simulink model "Ctrl_WT_openPI_IMC"  (R2019b)
settings: Solver=ode23tb  StartTime=0.0  StopTime=20  MaxStep=1/60  RelTol=1e-4  AbsTol=1e-3  EnableMultiTasking=on
InitFcn:
  | xInitial = init_power_wind_ig;
values from neighbouring files (symbols this model uses):
  GDes = tf(1,[0.2/n 1])^n    [lin_WT.m]
  GProc = zpk_min(1,1)    [lin_WT.m]
undefined symbols (not defined in the file or in its folder): D1, Delta, F, find_system, Fnom, gcbh, H, Llr, Lls, p, Pnom, Rr, Rs, sps_rtmsupport, Vnom
libraries: powerlib x14, cstblocks x13, powerlib_meascontrol x4, re_lib x1
settings Model: PauseTimes=15  ExtModeAutoUpdateStatusClock=off  Creator=MathWorks  LastModifiedBy=estuser04
settings SolverCC: AutoScaleAbsTol=off  SolverResetMethod=Robust
settings DataIOCC: LimitDataPoints=on  SaveFormat=Array  SignalLoggingSaveFormat=ModelDataLogs  SaveOutput=off  SaveTime=off  ReturnWorkspaceOutputs=off  SignalLoggingName=logsOut
settings OptimizationCC: BlockReduction=off  DefaultParameterBehavior=Inlined  BufferReuse=off  ExpressionDepthLimit=2147483647  InitFltsAndDblsToZero=on  LifeSpan=inf
settings DebuggingCC: UnderspecifiedInitializationDetection=Classic  MergeDetectMultiDrivingBlocksExec=none  CheckExecutionContextPreStartOutputMsg=on  CheckExecutionContextRuntimeOutputMsg=on  SignalResolutionControl=TryResolveAllWithWarning  SolverPrmCheckMsg=warning  MultiTaskDSMMsg=warning  MultiTaskCondExecSysMsg=none  FcnCallInpInsideContextMsg=warning  StateNameClashWarn=warning  InitInArrayFormatMsg=none  SFUnexpectedBacktrackingDiag=warning  SFNoUnconditionalDefaultTransitionDiag=warning  SFExecutionAtInitializationDiag=none  ArithmeticOperatorsInVariantConditions=warning
settings HardwareCC: ProdBitPerPointer=32  ProdBitPerSizeT=32  ProdBitPerPtrDiffT=32  ProdLargestAtomicFloat=None  ProdIntDivRoundTo=Undefined  ProdEndianess=Unspecified  ProdWordSize=32  ProdHWDeviceType=32-bit Generic
settings ModelReferenceCC: PropagateSignalLabelsOutOfModel=off
settings SFSimCC: SimUseLocalCustomCode=off  CustomCodeUndefinedFunction=UseInterfaceOnly
settings RTWCC: RTWUseLocalCustomCode=off
settings CodeAppCC: StateflowObjectComments=on
settings GRTTargetCC: TargetLangStandard=C89/C90 (ANSI)  GeneratePreprocessorConditionals=Disable all  CombineOutputUpdateFcns=off  GRTInterface=on
settings ConfigComp: CovMetricSettings=dw  CovHtmlReporting=on  CovSaveCumulativeToWorkspaceVar=on  CovSaveSingleToWorkspaceVar=on  CovExternalEMLEnable=off  CovSFcnEnable=off
settings SimscapeCC: SimscapeNormalizeSystem=off

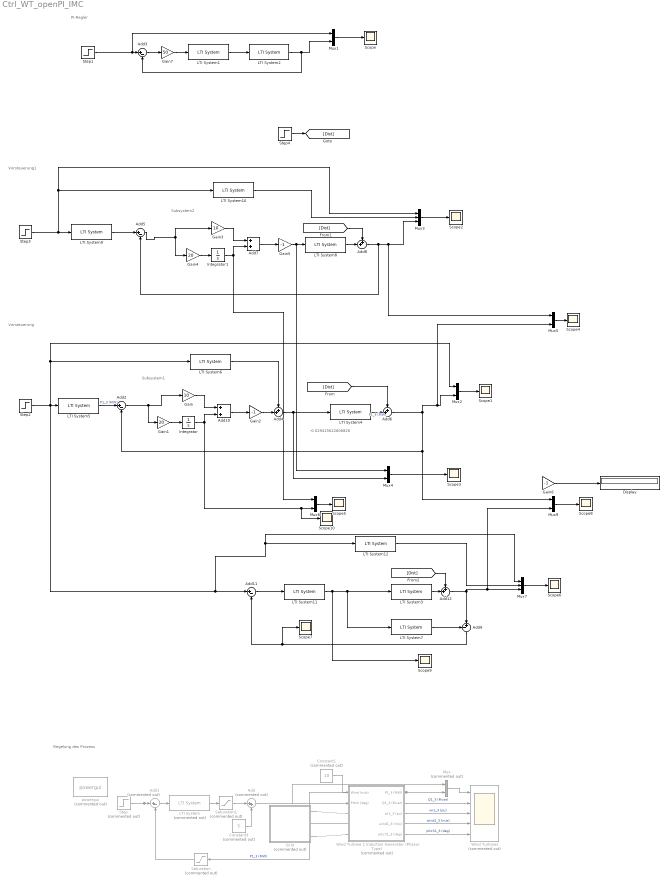
== system Ctrl_WT_openPI_IMC ==
  note: -0.029415622606826
  note: Subsystem2
  note: Subsystem1
  note: Regelung des Prozess
  note: PI-Regler
  note: Vorsteuerung
  note: Vorsteuerung1
  " Wind Turbines" : Scope  Commented=on  NumInputPorts=5
  Add : Sum  Commented=on  Inputs=|++
  Add1 : Sum  Commented=on  Inputs=|+-
  Add10 : Sum
  Add{2..3,5,11} (4 alike) : Sum  Inputs=|+-
  Add{4,6,8,12} (4 alike) : Sum  Inputs=++|
  Add7 : Sum
  Add9 : Sum  Inputs=-+|
  Constant1 : Constant  Commented=on  Value=10
  Constant3 : Constant  Commented=on  Value=5
  Display : Display
  Gain : Gain  Gain=10
  Gain1 : Gain  Gain=20
  Gain2 : Gain  Gain=-1
  Gain3 : Gain  Gain=10
  Gain4 : Gain  Gain=20
  Gain5 : Gain  Gain=-1
  Gain6 : Gain  Gain=-1
  Gain7 : Gain  Gain=50
  Grid : Subsystem  Commented=on
  Integrator : Integrator
  Integrator1 : Integrator
  LTI System : cstblocks/LTI System  Commented=on  sys=Creg  IC=[]
  LTI System1 : cstblocks/LTI System  sys=GRegPI  IC=[]
  LTI System10 : cstblocks/LTI System  sys=GDes  IC=[]
  LTI System11 : cstblocks/LTI System  sys=GDes/GProc  IC=[]
  LTI System12 : cstblocks/LTI System  sys=GDes  IC=[]
  LTI System2 : cstblocks/LTI System  sys=GProc  IC=[]
  LTI System{3..4,7..8} (4 alike) : cstblocks/LTI System  sys=GProcReal  IC=[]
  LTI System5 : cstblocks/LTI System  sys=GDes  IC=[]
  LTI System6 : cstblocks/LTI System  sys=GFF2  IC=[]
  LTI System9 : cstblocks/LTI System  sys=GFF  IC=[]
  Mux : Mux  Commented=on  Inputs=2
  Mux{1..2,4..6,9} (6 alike) : Mux  Inputs=2
  Mux3 : Mux  Inputs=3
  Mux7 : Mux  Inputs=3
  Saturation : Saturate  Commented=on  UpperLimit=1.5  LowerLimit=0.5
  Saturation1 : Saturate  Commented=on  UpperLimit=20  LowerLimit=-5
  Scope{,1..10} (11 alike) : Scope
  Step : Step  Commented=on  Time=5  Before=0.85  After=0.7  SampleTime=0
  Step1 : Step  Time=5  SampleTime=0
  Step2 : Step  Time=5  SampleTime=0
  Step3 : Step  Time=5  SampleTime=0
  Step4 : Step  Time=8  After=0  SampleTime=0
  Wind Turbine 1 Induction Generator (Phasor Type) : Subsystem  Commented=on  DialogController=POWERSYS.PowerSysDialog  LoadFcn=sps_rtmsupport('LoadFcn',gcbh); %find_system(gcs,'FollowLinks', 'on', 'LookUnderMasks', 'all');  StartFcn=sps_rtmsupport('StartFcn',gcbh);  StopFcn=sps_rtmsupport('StopFcn',gcbh);  mask(Wind Turbine Induction Generator (Phasor Type)){ExternalTm=off, nom=[2*1.5e6/0.9 575 60], sta=[ 0.004843 0.1248], rot=[ 0.004377 0.1791], Lm=6.77, mec=[5.04 0.01 3], init=[ -0.01,0   0,0,0   0,0,0 ], pitch_angle=0, Pmec=2*1.5e6, wind_base=9, speed_nom=1, P_wind_base=1, K_pitch_gain=[5 25], pitch_max=45, pitch_rate=2}
      mask prompts: ExternalTm "External turbine (Tm mechanical torque input)"; nom "Nominal power, line-to-line voltage, frequency [Pn(VA), Vn(Vrms), fn(Hz)]:"; sta "Stator [Rs, Lls] (pu):"; rot "Rotor [Rr', Llr'] (pu):"; Lm "Magnetizing inductance Lm (pu):"; mec "Inertia constant, friction factor, and pairs of poles: [H(s), F(pu), p]"; init "Initial conditions [s, th(deg), ias, ibs, ics (pu), ph_as, ph_bs, ph_cs (pu)]:"; pitch_angle "Pitch angle beta used to display characteristics (beta >=0)  (deg):"; Pmec "Nominal wind turbine mechanical output power (W):"; wind_base "Base wind speed (m/s):"; speed_nom "Base rotational speed (pu of base generator speed):"; P_wind_base "Maximum power at base wind speed (pu of nominal mechanical power):"; K_pitch_gain "Pitch angle controller gain: [Kp Ki]"; pitch_max "Maximum pitch angle (deg):"; pitch_rate "Maximum rate of change of pitch angle (deg/s):"
      mask help: Implements a phasor model of a squirrel-cage induction generator driven by a wind turbine.
      mask init:
      | [Pnom,Vnom,Fnom,Rs,Lls,Rr,Llr,H,p,F,Wind_On,FACTSroot] = WindTurbineIndGenInit (nom,sta,rot,mec,ExternalTm,wind_base,gcbh);
      settings: CopyFcn=sps_rtmsupport('CopyFcn',gcbh);  DeleteFcn=sps_rtmsupport('DeleteFcn',gcbh);  UndoDeleteFcn=sps_rtmsupport('UndoDeleteFcn',gcbh);  ModelCloseFcn=sps_rtmsupport('ModelCloseFcn',gcbh);  PreSaveFcn=sps_rtmsupport('PreSaveFcn',gcbh);  PostSaveFcn=sps_rtmsupport('PostSaveFcn',gcbh);  NameChangeFcn=sps_rtmsupport('NameChangeFcn',gcbh);  PreCopyFcn=sps_rtmsupport('PreCopyFcn',gcbh);  OpenFcn=sps_rtmsupport('OpenFcn',gcbh, [1]);  CloseFcn=sps_rtmsupport('CloseFcn',gcbh);  PreDeleteFcn=sps_rtmsupport('PreDeleteFcn',gcbh);
      mask Help: helpview(psbhelp);
      mask Callback ExternalTm: WindTurbineIndGenCback(gcbh);
      mask DialogControl generatordata Prompt: Generator
      mask DialogControl Turbine Prompt: Turbine
      mask DialogControl display Prompt: Display wind turbine power characteristics
      mask DialogControl display Callback: WindTurbineIndGenDisplay(gcbh);
  powergui : powerlib/powergui  Priority=2  Commented=on  SimulationMode=Phasor  SampleTime=0  frequency=60  Iterations=50  frequencyindice=60  Pbase=100e6  ErrMax=1e-4  UnitsV=kV  UnitsW=MW  buscounter=0  FunctionMessages=off  echomessages=off  EnableUseOfTLC=off  CurrentSourceSwitches=off  DisableSnubberDevices=off  DisableRonSwitches=off  DisableVfSwitches=off  DisplayEquations=off  AutomaticDiscreteSolvers=off  SolverType=Tustin  Interpol=off  ExternalGateDelay=off  methode=off  Ts=0  x0status=blocks  SPID=off  SwTol=0  HookPort=off  NonlinearTolerance=1e-4  nMaxIteration=100  ContinueOnMaxIteration=off  RestoreLinks=no  ResistiveCurrentMeasurement=off  Frange=[0:2:500]  Ylog=off  Xlog=off  ShowGrid=off  save=off  variable=ZData  structure=0  ZoomFFT=on  StartTime=0.0  cycles=1  DisplayStyle=1  fundamental=60  FreqAxis=off  MaxFrequency=1000  frequencyindicesteady=1  RmsSteady=1  display=off
      settings: SourceProductName=Simscape Electrical
  wires:
  Add/1 -> Wind Turbine 1 Induction Generator (Phasor Type)/2(Pitch (deg))
  Wind Turbine 1 Induction Generator (Phasor Type)/1(P1_3 (MW)) -> Mux/2, Saturation/1  "P1_3 (MW)"
  Wind Turbine 1 Induction Generator (Phasor Type)/4(wind1_3 (m/s)) -> " Wind Turbines"/4  "wind1_3 (m/s)"
  Wind Turbine 1 Induction Generator (Phasor Type)/3(wr1_3 (pu)) -> " Wind Turbines"/3  "wr1_3 (pu)"
  Constant1/1 -> Wind Turbine 1 Induction Generator (Phasor Type)/1("Wind (m/s) ")
  Wind Turbine 1 Induction Generator (Phasor Type)/2(Q1_3 (Mvar)) -> " Wind Turbines"/2  "Q1_3 (Mvar)"
  Wind Turbine 1 Induction Generator (Phasor Type)/5(pitch1_3 (deg)) -> " Wind Turbines"/5  "pitch1_3 (deg)"
  LTI System/1 -> Saturation1/1
  Add1/1 -> LTI System/1
  Saturation/1 -> Add1/2
  Step/1 -> Mux/1, Add1/1
  Saturation1/1 -> Add/1
  Constant3/1 -> Add/2
  Mux/1 -> " Wind Turbines"/1
  Mux1/1 -> Scope/1
  Step1/1 -> Add3/1, Mux1/1
  Add3/1 -> Gain7/1
  LTI System2/1 -> Mux1/2, Add3/2
  LTI System1/1 -> LTI System2/1
  LTI System4/1 -> Add6/2  "P1_3 (MW)"
  Mux2/1 -> Scope1/1
  LTI System5/1 -> Add2/1  "P1_3 (MW)"
  Gain2/1 -> Add4/2
  LTI System6/1 -> Add4/1
  Gain5/1 -> Mux4/1, LTI System8/1
  LTI System8/1 -> Add8/2
  Step3/1 -> LTI System9/1, LTI System10/1, Mux3/1
  Mux3/1 -> Scope2/1
  LTI System9/1 -> Add5/1
  LTI System10/1 -> Mux3/2
  Mux4/1 -> Scope3/1
  Add6/1 -> Mux9/1, Add2/2, Mux5/2, Mux2/2
  Add2/1 -> Gain1/1, Gain/1
  Integrator/1 -> Scope10/1, Mux6/2, Add10/2
  Add10/1 -> Gain2/1
  Gain/1 -> Add10/1
  Gain1/1 -> Integrator/1
  Gain4/1 -> Integrator1/1
  Gain3/1 -> Add7/1
  Add7/1 -> Gain5/1
  Integrator1/1 -> Mux6/1, Add7/2
  Add5/1 -> Gain4/1, Gain3/1
  Add8/1 -> Mux5/1, Mux3/3, Add5/2
  Step4/1 -> [Dist]
  [Dist] -> Add6/1
  [Dist] -> Add8/1
  Mux5/1 -> Scope4/1
  Mux6/1 -> Scope5/1
  Gain6/1 -> Display/1
  Mux9/1 -> Scope8/1
  LTI System7/1 -> Add9/1
  LTI System3/1 -> Add12/2
  Add11/1 -> LTI System11/1
  Add9/1 -> Scope7/1, Add11/2
  Mux7/1 -> Scope6/1
  LTI System12/1 -> Mux7/2
  Add12/1 -> Add9/2, Mux9/2, Mux7/3
  Step2/1 -> Add11/1, Mux7/1, LTI System12/1, LTI System5/1, Mux2/1, LTI System6/1
  [Dist] -> Add12/1
  LTI System11/1 -> LTI System3/1, LTI System7/1, Scope9/1
  Add4/1 -> LTI System4/1, Mux4/2
  Gain7/1 -> LTI System1/1
  connections:
  Grid/RConn1 -- Wind Turbine 1 Induction Generator (Phasor Type)/LConn1
  Wind Turbine 1 Induction Generator (Phasor Type)/LConn2 -- Grid/RConn2
  Grid/RConn3 -- Wind Turbine 1 Induction Generator (Phasor Type)/LConn3

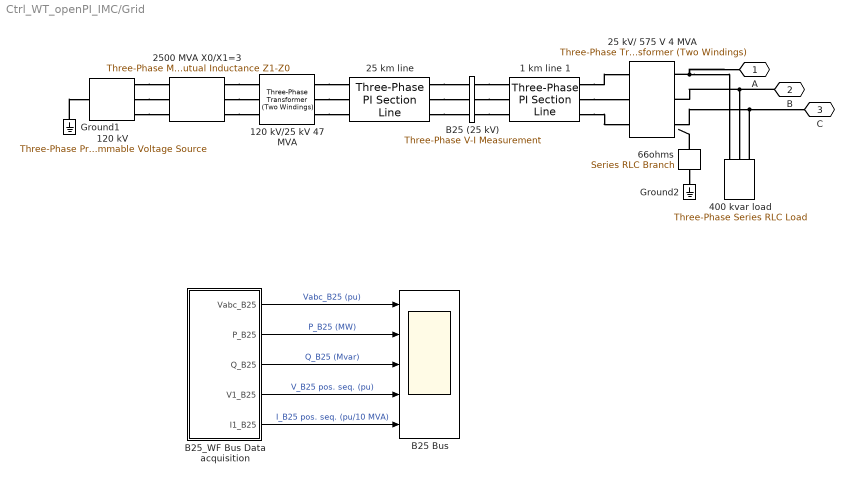
== system Ctrl_WT_openPI_IMC/Grid ==
  "1 km line 1 " : powerlib/Elements/Three-Phase PI Section Line  LConnTagsString=a|b|c  RConnTagsString=A|B|C  Frequency=60  Resistances=[0.1153 0.413]  Inductances=[1.05e-3 3.32e-3]  Capacitances=[11.33e-009 5.01e-009]  Length=1
      settings: SourceProductName=Simscape Electrical
  120 kV : powerlib/Electrical Sources/Three-Phase Programmable Voltage Source  PositiveSequence=[120e3 0 60]  VariationEntity=None  VariationType=Table of time-amplitude pairs  VariationTypeAlt=Step  VariationStep=-0.15  VariationRate=10  VariationMagnitude=0.3  VariationFrequency=2  VariationTiming=[5 5.5]  VariationPhaseA=off  Amplitudes="[1.0  0.5  1.0 ]"  TimeValues="[0  10  10.1]"  HarmonicGeneration=off  HarmonicA=[1 -0.1 0 1]  HarmonicB=[2 0.15 35 2]  Timing="[5  5.5]"  BusType=swing  Pref=1e3  Qref=0  Qmin=-inf  Qmax=inf
      settings: SourceProductName=Simscape Electrical
  120 kV/25 kV 47 MVA : powerlib/Elements/Three-Phase Transformer (Two Windings)  Winding1Connection=Yg  Winding2Connection=Delta (D1)  CoreType=Three single-phase transformers  SetSaturation=off  Hysteresis=off  DataFile='basic_model'  SetInitialFlux=off  Measurements=None  UNITS=pu  NominalPower=[47e6 60 ]  Winding1="[ 120e3  0.08/30   0.08 ]"  Winding2="[ 25e3  0.08/30  0.08]"  Rm=500  Lm=500  L0=0.5  Saturation="[ 0,0  ;  0.005,1.2  ;  1.0,1.4 ]"  InitialFluxes=[ 0.8 , -0.8 , 0.7 ]  BreakLoop=off  DiscreteSolver=Trapezoidal iterative  DataType=off  TransfoNumber=0
      settings: SourceProductName=Simscape Electrical
  25 kV/ 575 V 4 MVA : powerlib/Elements/Three-Phase Transformer (Two Windings)  Winding1Connection=Yg  Winding2Connection=Yn  CoreType=Three single-phase transformers  SetSaturation=off  Hysteresis=off  DataFile='hysteresis'  SetInitialFlux=off  Measurements=None  UNITS=pu  NominalPower="[4e6  60]"  Winding1=[25e3 , 0.025/30 , 0.025]  Winding2=[ 575, 0.025/30 , 0.025]  Rm=500  Lm=inf  L0=0.5  Saturation=[ 0,0 ; 0.0024,1.2 ; 1.0,1.52 ]  InitialFluxes=[ 0.8 , -0.8 , 0.7 ]  BreakLoop=off  DiscreteSolver=Trapezoidal iterative  DataType=off  TransfoNumber=0
      settings: SourceProductName=Simscape Electrical
  25 km line : powerlib/Elements/Three-Phase PI Section Line  LConnTagsString=a|b|c  RConnTagsString=A|B|C  Frequency=60  Resistances=[0.1153 0.413]  Inductances=[1.05e-3 3.32e-3]  Capacitances=[11.33e-009 5.01e-009]  Length=25
      settings: SourceProductName=Simscape Electrical
  2500 MVA X0/X1=3 : powerlib/Elements/Three-Phase Mutual Inductance Z1-Z0  LConnTagsString=a|b|c  RConnTagsString=A|B|C  PositiveSequence="[0.1  1.0/(2*pi*60)] *120e3^2/2500e6"  ZeroSequence="[0.3  3.0/(2*pi*60)] *120e3^2/2500e6"
      settings: SourceProductName=Simscape Electrical  SourceProductBaseCode=PS
  400 kvar load : powerlib/Elements/Three-Phase Series RLC Load  LConnTagsString=A|B|C  Configuration=Delta  NominalVoltage=575  Vabc=[1e3 1e3 1e3]  Vabcp=[1e3 1e3 1e3]  NominalFrequency=60  UnbalancedPower=off  ActivePower=0  InductivePower=0  CapacitivePower=400e3  Pabc=[10e3 9e3 11e3]  QLabc=[100 90 110]  QCabc=[100 90 110]  Pabcp=[10e3 9e3 11e3]  QLabcp=[100 90 110]  QCabcp=[100 90 110]  Measurements=None  LoadType=constant Z
      settings: SourceProductName=Simscape Electrical
  "66ohms " : powerlib/Elements/Series RLC Branch  LConnTagsString=__new0  RConnTagsString=__new0  BranchType=R  Resistance=66  Inductance=1.0  SetiL0=off  InitialCurrent=0  Capacitance=1.0  Setx0=off  InitialVoltage=0  Measurements=None
      settings: SourceProductName=Simscape Electrical
  B25 (25 kV) : powerlib/Measurements/Three-Phase V-I Measurement  VoltageMeasurement=phase-to-ground  SetLabelV=on  LabelV=Vabc_B25  Vpu=on  VpuLL=off  CurrentMeasurement=yes  SetLabelI=on  LabelI=Iabc_B25  Ipu=on  Pbase=10e6  Vbase=25e3  OutputType=Complex  PhasorSimulation=on  PSBequivalent=0
      settings: SourceProductName=Simscape Electrical
  B25 Bus : Scope  NumInputPorts=5
  B25_WF Bus Data acquisition : Subsystem
  Ground1 : powerlib/Elements/Ground  LConnTagsString=a
      settings: SourceProductName=Simscape Electrical
  Ground2 : powerlib/Elements/Ground  LConnTagsString=a
      settings: SourceProductName=Simscape Electrical
  A : PMIOPort  Side=Right
  B : PMIOPort  Port=2  Side=Right
  C : PMIOPort  Port=3  Side=Right
  wires:
  B25_WF Bus Data acquisition/5(I1_B25) -> B25 Bus/5  "I_B25 pos. seq. (pu/10 MVA)"
  B25_WF Bus Data acquisition/2(P_B25) -> B25 Bus/2  "P_B25 (MW)"
  B25_WF Bus Data acquisition/1("Vabc_B25 ") -> B25 Bus/1  "Vabc_B25 (pu)"
  B25_WF Bus Data acquisition/3(Q_B25) -> B25 Bus/3  "Q_B25 (Mvar)"
  B25_WF Bus Data acquisition/4(V1_B25) -> B25 Bus/4  "V_B25 pos. seq. (pu)"
  connections:
  "66ohms "/RConn1 -- Ground2/LConn1
  B25 (25 kV)/RConn3 -- "1 km line 1 "/LConn3
  "1 km line 1 "/RConn2 -- 25 kV/ 575 V 4 MVA/LConn2
  Ground1/LConn1 -- 120 kV/LConn1
  400 kvar load/LConn3 -- 25 kV/ 575 V 4 MVA/RConn3 -- C/RConn1
  "1 km line 1 "/RConn1 -- 25 kV/ 575 V 4 MVA/LConn1
  "1 km line 1 "/RConn3 -- 25 kV/ 575 V 4 MVA/LConn3
  "66ohms "/LConn1 -- ?
  25 km line/RConn1 -- B25 (25 kV)/LConn1
  120 kV/RConn1 -- 2500 MVA X0/X1=3/LConn1
  25 km line/RConn3 -- B25 (25 kV)/LConn3
  120 kV/25 kV 47 MVA/RConn3 -- 25 km line/LConn3
  25 km line/RConn2 -- B25 (25 kV)/LConn2
  2500 MVA X0/X1=3/RConn3 -- 120 kV/25 kV 47 MVA/LConn3
  2500 MVA X0/X1=3/RConn1 -- 120 kV/25 kV 47 MVA/LConn1
  25 kV/ 575 V 4 MVA/RConn1 -- 400 kvar load/LConn1 -- A/RConn1
  120 kV/RConn3 -- 2500 MVA X0/X1=3/LConn3
  B/RConn1 -- 400 kvar load/LConn2 -- 25 kV/ 575 V 4 MVA/RConn2
  120 kV/25 kV 47 MVA/RConn2 -- 25 km line/LConn2
  2500 MVA X0/X1=3/RConn2 -- 120 kV/25 kV 47 MVA/LConn2
  B25 (25 kV)/RConn2 -- "1 km line 1 "/LConn2
  120 kV/25 kV 47 MVA/RConn1 -- 25 km line/LConn1
  B25 (25 kV)/RConn1 -- "1 km line 1 "/LConn1
  120 kV/RConn2 -- 2500 MVA X0/X1=3/LConn2

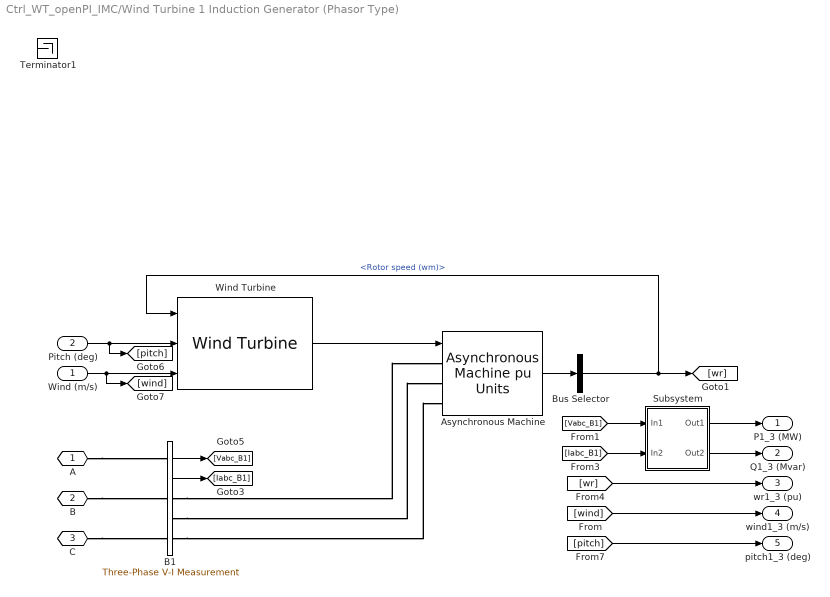
== system Ctrl_WT_openPI_IMC/Wind Turbine 1 Induction Generator (Phasor Type) ==
  "Wind (m/s) " : Inport
  Pitch (deg) : Inport  Port=2
  Asynchronous Machine : powerlib/Machines/Asynchronous Machine pu Units  RotorType=Squirrel-cage  PresetModel=No  MechanicalLoad=Torque Tm  ShowDetailedParameters=on  ReferenceFrame=Rotor  Units=pu  MeasurementBus=off  NominalParameters=[ Pnom Vnom Fnom ]  Stator=[ Rs Lls]  Rotor=[ Rr Llr]  Cage1=[0.01909 0.0397]  Cage2=[0.01909 0.0397]  Lm=Lm  Mechanical=[H F p]  PolePairs=3  InitialConditions=init  SimulateSaturation=off  Saturation=[ 0 0 ; 0 0 ]  LoadFlowParameters=0  TsPowergui=0  TsBlock=-1  IterativeModel=Forward Euler  IterativeDiscreteModel=Trapezoidal non iterative  Pmec=0
      settings: SourceProductName=Simscape Electrical  SourceProductBaseCode=PS
  B1 : powerlib/Measurements/Three-Phase V-I Measurement  VoltageMeasurement=phase-to-ground  SetLabelV=off  LabelV=Vabc_B1  Vpu=on  VpuLL=off  CurrentMeasurement=yes  SetLabelI=off  LabelI=Iabc_Beol  Ipu=on  Pbase=Pnom  Vbase=Vnom  OutputType=Complex  PhasorSimulation=on  PSBequivalent=0
      settings: SourceProductName=Simscape Electrical
  Bus Selector : BusSelector  OutputSignals=Mechanical.Rotor speed (wm)
  Subsystem : Subsystem
  Terminator1 : Terminator
  Wind Turbine : re_lib/Wind Generation/Wind Turbine  Pnom=Pmec  Pelec_base=Pnom  wind_base=wind_base  P_wind_base=P_wind_base  speed_nom=speed_nom  pitch_angle=0  c1_c6="[0.51763          116          0.4            5           21     0.006795]"  cp_nom=0.48  lambda_nom=8.1
      settings: SourceProductName=Simscape Electrical  SourceProductBaseCode=PS
  A : PMIOPort  Side=Left
  B : PMIOPort  Port=2  Side=Left
  C : PMIOPort  Port=3  Side=Left
  P1_3 (MW) : Outport  VectorParamsAs1DForOutWhenUnconnected=off
  Q1_3 (Mvar) : Outport  Port=2  VectorParamsAs1DForOutWhenUnconnected=off
  wr1_3 (pu) : Outport  Port=3  VectorParamsAs1DForOutWhenUnconnected=off
  wind1_3 (m/s) : Outport  Port=4  VectorParamsAs1DForOutWhenUnconnected=off
  pitch1_3 (deg) : Outport  Port=5  VectorParamsAs1DForOutWhenUnconnected=off
  wires:
  Asynchronous Machine/1 -> Bus Selector/1
  B1/2 -> [Iabc_B1]
  B1/1 -> [Vabc_B1]
  "Wind (m/s) "/1 -> Wind Turbine/3, [wind]
  Bus Selector/1 -> Wind Turbine/1, [wr]  "<Rotor speed (wm)>"
  Wind Turbine/1 -> Asynchronous Machine/1
  Pitch (deg)/1 -> [pitch], Wind Turbine/2
  [pitch] -> pitch1_3 (deg)/1
  [wind] -> wind1_3 (m/s)/1
  [wr] -> wr1_3 (pu)/1
  [Vabc_B1] -> Subsystem/1(In1)
  [Iabc_B1] -> Subsystem/2(In2)
  Subsystem/1(Out1) -> P1_3 (MW)/1
  Subsystem/2(Out2) -> Q1_3 (Mvar)/1
  connections:
  B/RConn1 -- B1/LConn2
  C/RConn1 -- B1/LConn3
  A/RConn1 -- B1/LConn1
  B1/RConn1 -- Asynchronous Machine/LConn1
  B1/RConn2 -- Asynchronous Machine/LConn2
  B1/RConn3 -- Asynchronous Machine/LConn3

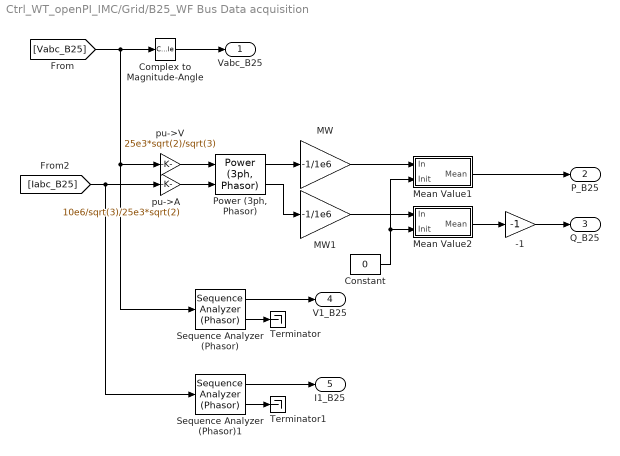
== system Ctrl_WT_openPI_IMC/Grid/B25_WF Bus Data acquisition ==
  -1 : Gain  Gain=-1  SaturateOnIntegerOverflow=on  OutDataTypeStr=Inherit: Same as input  ParamDataTypeStr=Inherit: Same as input
  "Complex to Magnitude-Angle " : ComplexToMagnitudeAngle  Output=Magnitude
  Constant : Constant  Value=0
  MW : Gain  Gain=-1/1e6  SaturateOnIntegerOverflow=on  OutDataTypeStr=Inherit: Same as input  ParamDataTypeStr=Inherit: Same as input
  MW1 : Gain  Gain=-1/1e6  SaturateOnIntegerOverflow=on  OutDataTypeStr=Inherit: Same as input  ParamDataTypeStr=Inherit: Same as input
  Mean Value1 : Subsystem  mask(Mean value){Period=1/60}
      mask prompts: Period "Averaging period (s):"
      mask help: This block uses the running window averaging technique to compute the mean value of the input signal over the specified period.
  Mean Value2 : Subsystem  mask(Mean value){Period=1/60}
      mask prompts: Period "Averaging period (s):"
      mask help: This block uses the running window averaging technique to compute the mean value of the input signal over the specified period.
  "Power (3ph, Phasor)" : powerlib_meascontrol/Measurements/Power (3ph, Phasor)
      settings: SourceProductName=Simscape Electrical  SourceProductBaseCode=PS
  Sequence Analyzer (Phasor) : powerlib_meascontrol/Measurements/Sequence Analyzer (Phasor)  seq=Positive
      settings: SourceProductName=Simscape Electrical  SourceProductBaseCode=PS
  Sequence Analyzer (Phasor)1 : powerlib_meascontrol/Measurements/Sequence Analyzer (Phasor)  seq=Positive
      settings: SourceProductName=Simscape Electrical  SourceProductBaseCode=PS
  Terminator : Terminator
  Terminator1 : Terminator
  pu->A : Gain  Gain=10e6/sqrt(3)/25e3*sqrt(2)  SaturateOnIntegerOverflow=on  OutDataTypeStr=Inherit: Same as input  ParamDataTypeStr=Inherit: Same as input
  pu->V : Gain  Gain=25e3*sqrt(2)/sqrt(3)  SaturateOnIntegerOverflow=on  OutDataTypeStr=Inherit: Same as input  ParamDataTypeStr=Inherit: Same as input
  "Vabc_B25 " : Outport  VectorParamsAs1DForOutWhenUnconnected=off
  P_B25 : Outport  Port=2  VectorParamsAs1DForOutWhenUnconnected=off
  Q_B25 : Outport  Port=3  VectorParamsAs1DForOutWhenUnconnected=off
  V1_B25 : Outport  Port=4  VectorParamsAs1DForOutWhenUnconnected=off
  I1_B25 : Outport  Port=5  VectorParamsAs1DForOutWhenUnconnected=off
  wires:
  pu->A/1 -> "Power (3ph, Phasor)"/2
  pu->V/1 -> "Power (3ph, Phasor)"/1
  "Power (3ph, Phasor)"/1 -> MW/1
  "Complex to Magnitude-Angle "/1 -> "Vabc_B25 "/1
  [Vabc_B25] -> Sequence Analyzer (Phasor)/1, pu->V/1, "Complex to Magnitude-Angle "/1
  [Iabc_B25] -> Sequence Analyzer (Phasor)1/1, pu->A/1
  MW/1 -> Mean Value1/1(In)
  MW1/1 -> Mean Value2/1(In)
  Constant/1 -> Mean Value1/2(Init), Mean Value2/2(Init)
  Mean Value1/1(Mean) -> P_B25/1
  Mean Value2/1(Mean) -> -1/1
  Sequence Analyzer (Phasor)/1 -> V1_B25/1
  Sequence Analyzer (Phasor)/2 -> Terminator/1
  Sequence Analyzer (Phasor)1/1 -> I1_B25/1
  Sequence Analyzer (Phasor)1/2 -> Terminator1/1
  -1/1 -> Q_B25/1
  "Power (3ph, Phasor)"/2 -> MW1/1

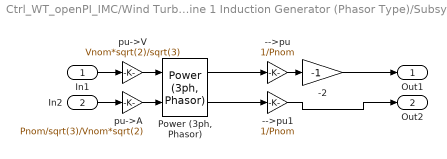
== system Ctrl_WT_openPI_IMC/Wind Turbine 1 Induction Generator (Phasor Type)/Subsystem ==
  In1 : Inport
  In2 : Inport  Port=2
  -->pu : Gain  Gain=1/Pnom  SaturateOnIntegerOverflow=on  OutDataTypeStr=Inherit: Same as input  ParamDataTypeStr=Inherit: Same as input
  -->pu1 : Gain  Gain=1/Pnom  SaturateOnIntegerOverflow=on  OutDataTypeStr=Inherit: Same as input  ParamDataTypeStr=Inherit: Same as input
  -2 : Gain  Gain=-1  SaturateOnIntegerOverflow=on  OutDataTypeStr=Inherit: Same as input  ParamDataTypeStr=Inherit: Same as input
  "Power (3ph, Phasor)" : powerlib_meascontrol/Measurements/Power (3ph, Phasor)
      settings: SourceProductName=Simscape Electrical  SourceProductBaseCode=PS
  pu->A : Gain  Gain=Pnom/sqrt(3)/Vnom*sqrt(2)  SaturateOnIntegerOverflow=on  OutDataTypeStr=Inherit: Same as input  ParamDataTypeStr=Inherit: Same as input
  pu->V : Gain  Gain=Vnom*sqrt(2)/sqrt(3)  SaturateOnIntegerOverflow=on  OutDataTypeStr=Inherit: Same as input  ParamDataTypeStr=Inherit: Same as input
  Out1 : Outport
  Out2 : Outport  Port=2
  wires:
  In2/1 -> pu->A/1
  -->pu/1 -> -2/1
  "Power (3ph, Phasor)"/1 -> -->pu/1
  pu->A/1 -> "Power (3ph, Phasor)"/2
  -2/1 -> Out1/1
  "Power (3ph, Phasor)"/2 -> -->pu1/1
  pu->V/1 -> "Power (3ph, Phasor)"/1
  In1/1 -> pu->V/1
  -->pu1/1 -> Out2/1

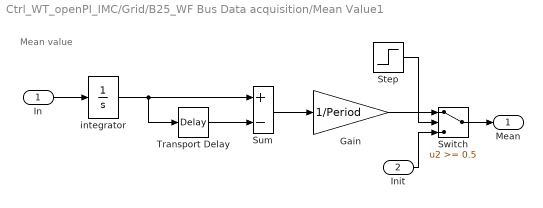
== system Ctrl_WT_openPI_IMC/Grid/B25_WF Bus Data acquisition/Mean Value1 ==
  note: Mean value
  In : Inport
  Init : Inport  Port=2
  Gain : Gain  Gain=1/Period  SaturateOnIntegerOverflow=on  OutDataTypeStr=Inherit: Same as input  ParamDataTypeStr=Inherit: Same as input
  Step : Step  Time=Period+eps  SampleTime=0
  Sum : Sum  Inputs=+-  SaturateOnIntegerOverflow=on  InputSameDT=on  OutDataTypeStr=Inherit: Same as first input
  Switch : Switch  Threshold=0.5  SaturateOnIntegerOverflow=on
  Transport Delay : TransportDelay  DelayTime=Period
  integrator : Integrator
  Mean : Outport  VectorParamsAs1DForOutWhenUnconnected=off
  wires:
  Transport Delay/1 -> Sum/2
  integrator/1 -> Transport Delay/1, Sum/1
  In/1 -> integrator/1
  Sum/1 -> Gain/1
  Gain/1 -> Switch/1
  Switch/1 -> Mean/1
  Step/1 -> Switch/2
  Init/1 -> Switch/3

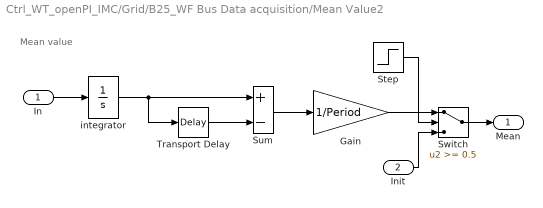
== system Ctrl_WT_openPI_IMC/Grid/B25_WF Bus Data acquisition/Mean Value2 ==
  note: Mean value
  In : Inport
  Init : Inport  Port=2
  Gain : Gain  Gain=1/Period  SaturateOnIntegerOverflow=on  OutDataTypeStr=Inherit: Same as input  ParamDataTypeStr=Inherit: Same as input
  Step : Step  Time=Period+eps  SampleTime=0
  Sum : Sum  Inputs=+-  SaturateOnIntegerOverflow=on  InputSameDT=on  OutDataTypeStr=Inherit: Same as first input
  Switch : Switch  Threshold=0.5  SaturateOnIntegerOverflow=on
  Transport Delay : TransportDelay  DelayTime=Period
  integrator : Integrator
  Mean : Outport  VectorParamsAs1DForOutWhenUnconnected=off
  wires:
  Init/1 -> Switch/3
  Step/1 -> Switch/2
  Switch/1 -> Mean/1
  Gain/1 -> Switch/1
  Sum/1 -> Gain/1
  In/1 -> integrator/1
  integrator/1 -> Sum/1, Transport Delay/1
  Transport Delay/1 -> Sum/2
